simulink model "realtimemodel"  (R2024b)
settings: Solver=ode5  StartTime=0.0  StopTime=5  FixedStep=0.001  RelTol=1e-3
undefined symbols (not defined in the file): DiscIntNeverNeededParam, feedback, filt, LQR, National_Instruments, PCIe, sens, sIn
libraries: sldrtlib x3, simulink x1
settings Model: SimulationMode=external  ExtModeTrigDuration=10001  Creator=surinihal  LastModifiedBy=surinihal
settings DataIOCC: ReturnWorkspaceOutputs=off
settings HardwareCC: ProdBitPerLong=64  ProdHWDeviceType=Intel->x86-64 (Linux 64)
settings RTWCC: Description=Simulink Desktop Real-Time  SystemTargetFile=sldrt.tlc  TemplateMakefile=sldrt.tmf  RTWCompilerOptimization=on
settings CodeAppCC: MaxIdLength=95
settings SimulinkDesktopRealTimeCC: TargetLibSuffix=_sldrt.a  TargetPreCompLibLocation=C:\Program Files\MATLAB\R2024b\toolbox\sldrt\lib\win64  ParMdlRefBuildCompliant=on

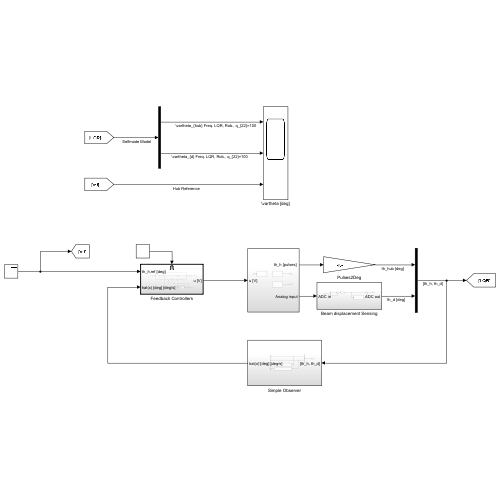
[thumbnail: Simulink's stored preview of the top-level diagram]
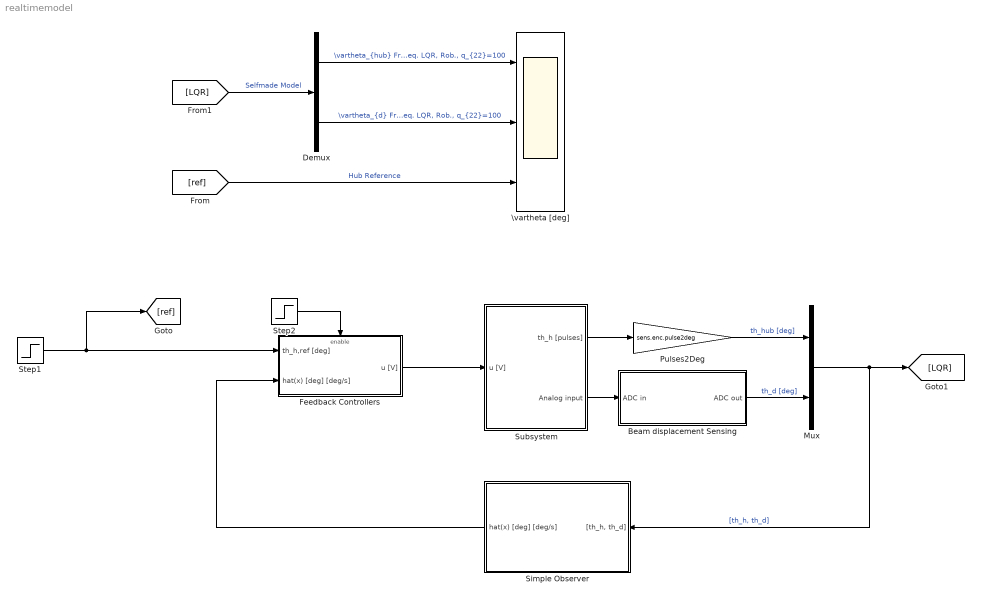
== system realtimemodel ==
  Beam displacement Sensing : Subsystem
  Demux : Demux  Outputs=2
  Feedback Controllers : Subsystem
  Mux : Mux  Inputs=2
  Pulses2Deg : Gain  Gain=sens.enc.pulse2deg
  Simple Observer : Subsystem
  Step1 : Step  Time=sIn.t1  After=sIn.position  SampleTime=0
  Step2 : Step  Time=sIn.t1  SampleTime=0
  Subsystem : Subsystem
  \vartheta [deg] : Scope  NumInputPorts=3
  wires:
  [ref] -> \vartheta [deg]/3  "Hub Reference"
  [LQR] -> Demux/1  "Selfmade Model"
  Demux/2 -> \vartheta [deg]/2  "\\vartheta_{d} Freq. LQR, Rob., q_{22}=100"
  Demux/1 -> \vartheta [deg]/1  "\\vartheta_{hub} Freq. LQR, Rob., q_{22}=100"
  Feedback Controllers/1(u [V]) -> Subsystem/1(u [V])
  Subsystem/2(Analog input) -> Beam displacement Sensing/1(ADC in)
  Subsystem/1("th_h [pulses] ") -> Pulses2Deg/1
  Simple Observer/1(hat(x) [deg] [deg/s]) -> Feedback Controllers/2(hat(x) [deg] [deg/s])
  Step2/1 -> Feedback Controllers/Enable
  Mux/1 -> Simple Observer/1("[th_h, th_d]"), [LQR]  "[th_h, th_d]"
  Step1/1 -> [ref], Feedback Controllers/1(th_h,ref [deg])
  Beam displacement Sensing/1(ADC out) -> Mux/2  "th_d [deg]"
  Pulses2Deg/1 -> Mux/1  "th_hub [deg]"

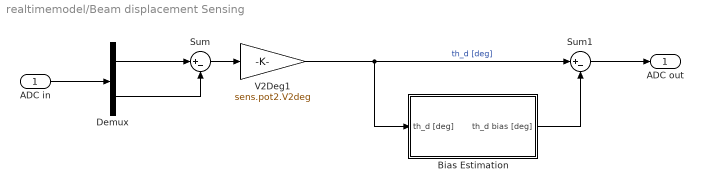
== system realtimemodel/Beam displacement Sensing ==
  ADC in : Inport
  Bias Estimation : Subsystem
  Demux : Demux  Outputs=2
  Sum : Sum  Inputs=|+-
  Sum1 : Sum  Inputs=|+-
  V2Deg1 : Gain  Gain=sens.pot2.V2deg
  ADC out : Outport
  wires:
  Bias Estimation/1(th_d bias [deg]) -> Sum1/2
  ADC in/1 -> Demux/1
  V2Deg1/1 -> Bias Estimation/1(th_d [deg]), Sum1/1  "th_d [deg]"
  Sum/1 -> V2Deg1/1
  Demux/2 -> Sum/2
  Demux/1 -> Sum/1
  Sum1/1 -> ADC out/1

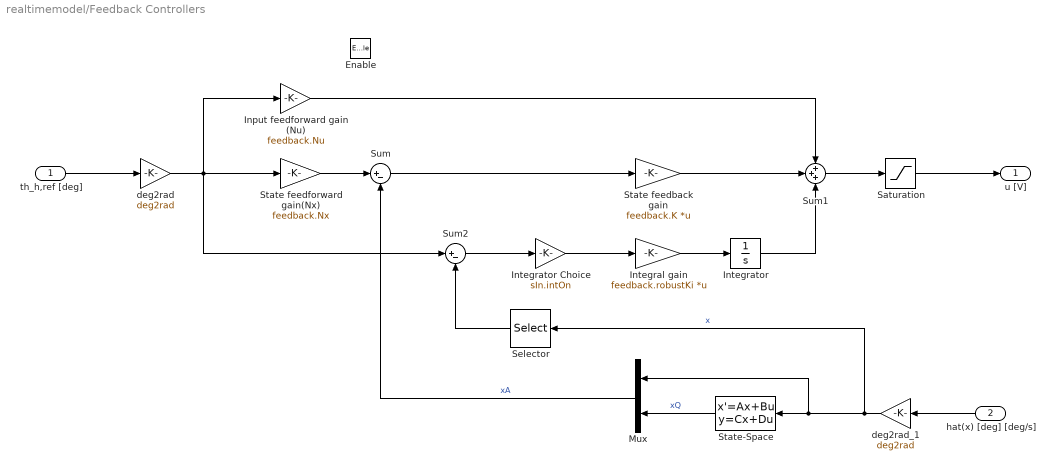
== system realtimemodel/Feedback Controllers ==
  th_h,ref [deg] : Inport
  hat(x) [deg] [deg/s] : Inport  Port=2
  Enable : EnablePort
  Input feedforward gain (Nu) : Gain  Gain=feedback.Nu
  Integral gain : Gain  Gain=feedback.robustKi  Multiplication=Matrix(K*u)
  Integrator : Integrator
  Integrator Choice : Gain  Gain=sIn.intOn
  Mux : Mux  Inputs=2
  Saturation : Saturate  UpperLimit=10  LowerLimit=-10
  Selector : Selector  InputPortWidth=4  IndexOptions=Index vector (dialog)  Indices=1  OutputSizes=1
  State feedback gain : Gain  Gain=feedback.K  Multiplication=Matrix(K*u)
  State feedforward gain(Nx) : Gain  Gain=feedback.Nx
  State-Space : StateSpace  A=LQR.AQ  B=LQR.BQ  C=eye(2,2)  D=zeros(2,4)  InitialCondition=0
  Sum : Sum  Inputs=|+-
  Sum1 : Sum  Inputs=+++
  Sum2 : Sum  Inputs=|+-
  deg2rad : Gain  Gain=deg2rad
  deg2rad_1 : Gain  Gain=deg2rad
  u [V] : Outport
  wires:
  Integrator/1 -> Sum1/3
  Sum1/1 -> Saturation/1
  State feedback gain/1 -> Sum1/2
  Sum2/1 -> Integrator Choice/1
  Selector/1 -> Sum2/2
  Integral gain/1 -> Integrator/1
  Sum/1 -> State feedback gain/1
  State feedforward gain(Nx)/1 -> Sum/1
  Saturation/1 -> u [V]/1
  th_h,ref [deg]/1 -> deg2rad/1
  hat(x) [deg] [deg/s]/1 -> deg2rad_1/1
  Input feedforward gain (Nu)/1 -> Sum1/1
  deg2rad/1 -> Input feedforward gain (Nu)/1, State feedforward gain(Nx)/1, Sum2/1
  deg2rad_1/1 -> Selector/1, Mux/1, State-Space/1  "x"
  State-Space/1 -> Mux/2  "xQ"
  Mux/1 -> Sum/2  "xA"
  Integrator Choice/1 -> Integral gain/1

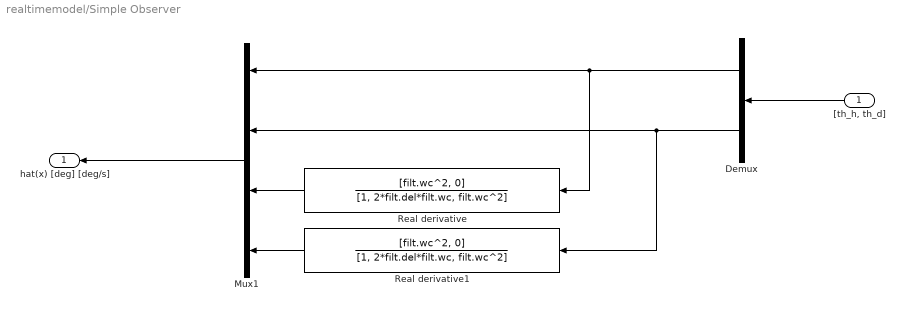
== system realtimemodel/Simple Observer ==
  "[th_h, th_d]" : Inport
  Demux : Demux  Outputs=2
  Mux1 : Mux
  Real derivative : TransferFcn  Numerator=[filt.wc^2, 0]  Denominator=[1, 2*filt.del*filt.wc, filt.wc^2]
  Real derivative1 : TransferFcn  Numerator=[filt.wc^2, 0]  Denominator=[1, 2*filt.del*filt.wc, filt.wc^2]
  hat(x) [deg] [deg/s] : Outport
  wires:
  Demux/1 -> Mux1/1, Real derivative/1
  Mux1/1 -> hat(x) [deg] [deg/s]/1
  "[th_h, th_d]"/1 -> Demux/1
  Real derivative/1 -> Mux1/3
  Demux/2 -> Real derivative1/1, Mux1/2
  Real derivative1/1 -> Mux1/4

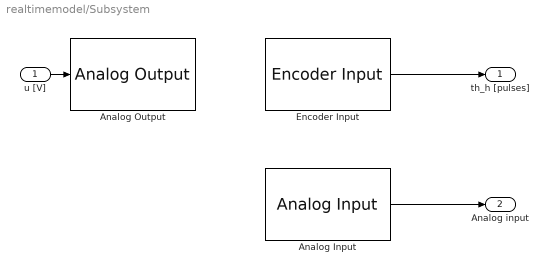
== system realtimemodel/Subsystem ==
  u [V] : Inport
  Analog Input : sldrtlib/Analog Input  SampleTime=-1  MaxMissedTicks=10  ShowMissedTicks=off  YieldWhenWaiting=off  DrvName=National_Instruments/PCIe-6321  DrvAddress=4294967295  DrvOptions=[0 0 0 2 0 0 0]  Channels=[3,4]  RangeMode=1  VoltRange=2  DataType=1
      settings: AttributesFormatString=National Instruments\nPCIe-6321 [auto]
  Analog Output : sldrtlib/Analog Output  SampleTime=-1  MaxMissedTicks=10  ShowMissedTicks=off  YieldWhenWaiting=off  DrvName=National_Instruments/PCIe-6321  DrvAddress=4294967295  DrvOptions=[0 0 0 2 0 0 0]  Channels=1  RangeMode=1  VoltRange=1  InitialValue=0  FinalValue=0
      settings: AttributesFormatString=National Instruments\nPCIe-6321 [auto]
  Encoder Input : sldrtlib/Encoder Input  SampleTime=-1  MaxMissedTicks=10  ShowMissedTicks=off  YieldWhenWaiting=off  DrvName=National_Instruments/PCIe-6321  DrvAddress=4294967295  DrvOptions=[0 0 0 2 0 0 0]  Channels=1  QuadMode=3  IndexPulse=1  InputFilter=Inf  DataType=1
      settings: AttributesFormatString=National Instruments\nPCIe-6321 [auto]
  "th_h [pulses] " : Outport
  Analog input : Outport  Port=2
  wires:
  u [V]/1 -> Analog Output/1
  Encoder Input/1 -> "th_h [pulses] "/1
  Analog Input/1 -> Analog input/1

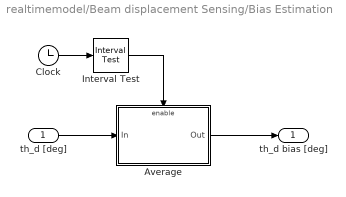
== system realtimemodel/Beam displacement Sensing/Bias Estimation ==
  th_d [deg] : Inport
  Average : Subsystem
  Clock : Clock
  Interval Test : simulink/Logic and Bit Operations/Interval Test  IntervalClosedRight=on  uplimit=sIn.t1  IntervalClosedLeft=on  lowlimit=sIn.t0  OutDataTypeStr=boolean
  th_d bias [deg] : Outport
  wires:
  Average/1(Out) -> th_d bias [deg]/1
  th_d [deg]/1 -> Average/1(In)
  Interval Test/1 -> Average/Enable
  Clock/1 -> Interval Test/1

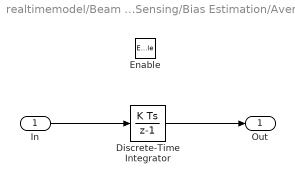
== system realtimemodel/Beam displacement Sensing/Bias Estimation/Average ==
  In : Inport
  Enable : EnablePort
  Discrete-Time Integrator : DiscreteIntegrator  gainval=1/(sIn.t1-sIn.t0)  SampleTime=-1  ICPrevOutput=DiscIntNeverNeededParam  ICPrevScaledInput=DiscIntNeverNeededParam
  Out : Outport
  wires:
  Discrete-Time Integrator/1 -> Out/1
  In/1 -> Discrete-Time Integrator/1
